simulink model "v2015a_Sensores"  (R2015a)
settings: Solver=ode45  SolverMode=SingleTasking  StartTime=0.0  StopTime=10.0  RelTol=1e-3
undefined symbols (not defined in the file): bias_mag, bias_sun, Eclipse, heading_mag, Mag_I, Pos_Sun_I, tilt_mag, v_I_S
libraries: simulink_extras x4, aerolibconvert2 x3, aerolibutil x2, aerolibtransform2 x2
settings Model: CovMetricSettings=dwe  CovHtmlReporting=off  covSaveCumulativeToWorkspaceVar=off  CovSaveSingleToWorkspaceVar=off  CovExternalEMLEnable=on  Creator=kakat  LastModifiedBy=kakat
settings DataIOCC: LimitDataPoints=off  SaveFormat=Dataset  ReturnWorkspaceOutputs=on
settings DebuggingCC: SFUnexpectedBacktrackingDiag=error  SFNoUnconditionalDefaultTransitionDiag=error
settings HardwareCC: ProdBitPerPointer=64  ProdLargestAtomicFloat=Float  ProdIntDivRoundTo=Zero  ProdEndianess=LittleEndian  ProdHWDeviceType=Specified
settings ModelReferenceCC: PropagateSignalLabelsOutOfModel=on
settings SFSimCC: SimUseLocalCustomCode=on
settings RTWCC: RTWUseLocalCustomCode=on
settings GRTTargetCC: TargetLangStandard=C99 (ISO)

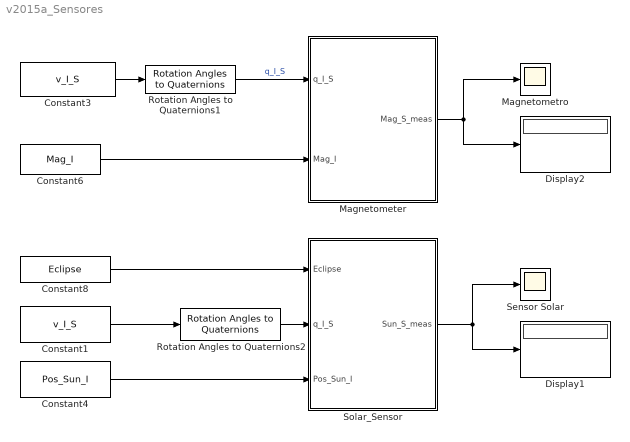
== system v2015a_Sensores ==
  Constant1 : Constant  Value=v_I_S
  Constant3 : Constant  Value=v_I_S
  Constant4 : Constant  Value=Pos_Sun_I
  Constant6 : Constant  Value=Mag_I
  Constant8 : Constant  Value=Eclipse
  Display1 : Display
  Display2 : Display
  Magnetometer : Subsystem
  Magnetometro : Scope
      settings: TimeRange=auto  MaxDataPoints=5000  SaveToWorkspace=off  YMin=-0.000045  YMax=0.000045  SampleTime=-1
  Rotation Angles to Quaternions1 : aerolibtransform2/Rotation Angles to Quaternions  rotationOrder=ZYX
  Rotation Angles to Quaternions2 : aerolibtransform2/Rotation Angles to Quaternions  rotationOrder=ZYX
  Sensor Solar : Scope
      settings: TimeRange=auto  MaxDataPoints=5000  SaveToWorkspace=off  SaveName=ScopeData  YMin=-182918141.73544  YMax=171344381.20005  SampleTime=-1
  Solar_Sensor : Subsystem
  wires:
  Constant3/1 -> Rotation Angles to Quaternions1/1
  Magnetometer/1(Mag_S_meas) -> Display2/1, Magnetometro/1
  Constant6/1 -> Magnetometer/2(Mag_I)
  Constant1/1 -> Rotation Angles to Quaternions2/1
  Rotation Angles to Quaternions2/1 -> Solar_Sensor/2(q_I_S)
  Solar_Sensor/1(Sun_S_meas) -> Display1/1, Sensor Solar/1
  Constant8/1 -> Solar_Sensor/1(Eclipse)
  Constant4/1 -> Solar_Sensor/3(Pos_Sun_I)
  Rotation Angles to Quaternions1/1 -> Magnetometer/1(q_I_S)  "q_I_S"

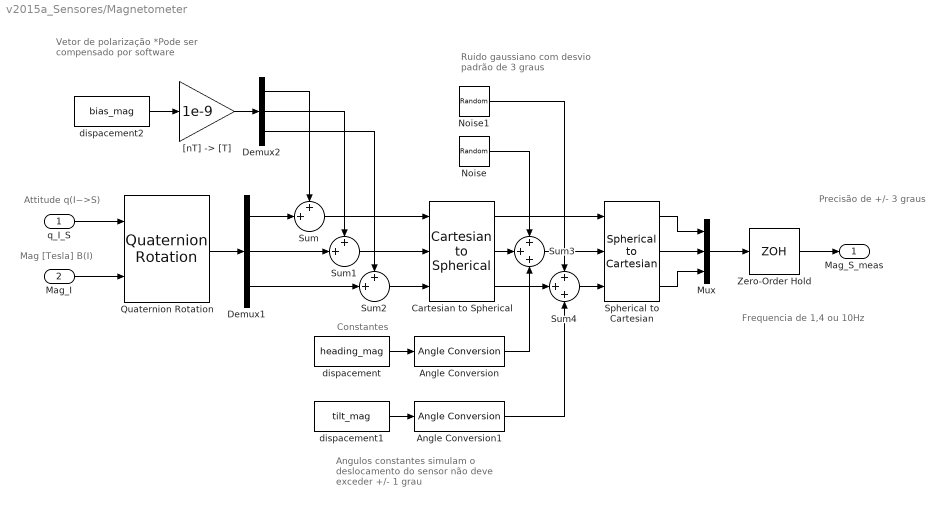
== system v2015a_Sensores/Magnetometer ==
  note: Attitude q(I−>S)
  note: Angulos constantes
      | simulam o deslocamento do sensor
      | não deve exceder +/- 1 grau
  note: Precisão de
      | +/- 3 graus
  note: Vetor de polarização
      | *Pode ser compensado
      | por software
  note: Frequencia de
      | 1,4 ou 10Hz
  note: Ruido gaussiano com
      | desvio padrão de 3 graus
  note: Constantes
  note: Mag [Tesla] B(I)
  q_I_S : Inport
  Mag_I : Inport  Port=2
  Angle Conversion : aerolibconvert2/Angle Conversion  IU=deg  OU=rad
  Angle Conversion1 : aerolibconvert2/Angle Conversion  IU=deg  OU=rad
  Cartesian to Spherical : simulink_extras/Transformations/Cartesian to Spherical
  Demux1 : Demux  Outputs=3
  Demux2 : Demux  Outputs=3
  Mux : Mux  Inputs=3
  Noise : RandomNumber  Variance=3  SampleTime=0.1
  Noise1 : RandomNumber  Variance=3  SampleTime=0.1
  Quaternion Rotation : aerolibutil/Quaternion Rotation
  Spherical to Cartesian : simulink_extras/Transformations/Spherical to Cartesian
  Sum : Sum  Inputs=++|
  Sum1 : Sum  Inputs=++|
  Sum2 : Sum  Inputs=++|
  Sum3 : Sum  Inputs=+++
  Sum4 : Sum  Inputs=+++
  Zero-Order Hold : ZeroOrderHold  SampleTime=.1
  "[nT] -> [T]" : Gain  Gain=1e-9
  dispacement : Constant  Value=heading_mag
  dispacement1 : Constant  Value=tilt_mag
  dispacement2 : Constant  Value=bias_mag
  Mag_S_meas : Outport
  wires:
  Quaternion Rotation/1 -> Demux1/1
  Mag_I/1 -> Quaternion Rotation/2
  Zero-Order Hold/1 -> Mag_S_meas/1
  Spherical to Cartesian/1 -> Mux/1
  Spherical to Cartesian/2 -> Mux/2
  dispacement1/1 -> Angle Conversion1/1
  Spherical to Cartesian/3 -> Mux/3
  Noise/1 -> Sum3/1
  Mux/1 -> Zero-Order Hold/1
  dispacement2/1 -> "[nT] -> [T]"/1
  dispacement/1 -> Angle Conversion/1
  Angle Conversion/1 -> Sum3/3
  Noise1/1 -> Sum4/1
  Demux1/1 -> Sum/2
  Angle Conversion1/1 -> Sum4/3
  q_I_S/1 -> Quaternion Rotation/1
  Cartesian to Spherical/2 -> Sum3/2
  Cartesian to Spherical/1 -> Spherical to Cartesian/1
  Sum3/1 -> Spherical to Cartesian/2
  Demux2/3 -> Sum2/1
  Sum4/1 -> Spherical to Cartesian/3
  Demux2/1 -> Sum/1
  Cartesian to Spherical/3 -> Sum4/2
  Demux1/3 -> Sum2/2
  Sum2/1 -> Cartesian to Spherical/3
  Sum/1 -> Cartesian to Spherical/1
  Demux1/2 -> Sum1/2
  Sum1/1 -> Cartesian to Spherical/2
  Demux2/2 -> Sum1/1
  "[nT] -> [T]"/1 -> Demux2/1

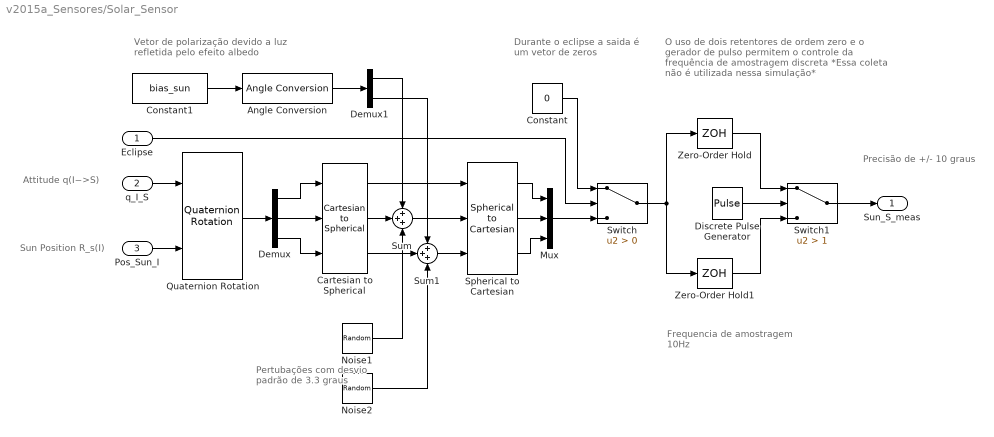
== system v2015a_Sensores/Solar_Sensor ==
  note: Sun Position R_s(I)
  note: O uso de dois retentores de ordem zero e o gerador de pulso permitem o controle da frequência de amostragem discreta
      |
      | *Essa coleta não é utilizada nessa simulação*
  note: Pertubações com desvio padrão de 3.3 graus
  note: Precisão de +/- 10 graus
  note: Vetor de polarização devido a luz refletida pelo efeito albedo
  note: Durante o eclipse a saida é um vetor de zeros
  note: Frequencia de amostragem 10Hz
  note: Attitude q(I−>S)
  Eclipse : Inport
  q_I_S : Inport  Port=2
  Pos_Sun_I : Inport  Port=3
  Angle Conversion : aerolibconvert2/Angle Conversion  IU=deg  OU=rad
  Cartesian to Spherical : simulink_extras/Transformations/Cartesian to Spherical
  Constant : Constant  Value=0
  Constant1 : Constant  Value=bias_sun
  Demux : Demux  Outputs=3
  Demux1 : Demux  Outputs=2
  Discrete Pulse Generator : DiscretePulseGenerator  Period=10  PulseWidth=5
  Mux : Mux  Inputs=3
  Noise1 : RandomNumber  SampleTime=0.1
  Noise2 : RandomNumber  SampleTime=0.1
  Quaternion Rotation : aerolibutil/Quaternion Rotation
  Spherical to Cartesian : simulink_extras/Transformations/Spherical to Cartesian
  Sum : Sum  Inputs=+++
  Sum1 : Sum  Inputs=+++
  Switch : Switch  Criteria=u2 > Threshold
      settings: LockScale=on
  Switch1 : Switch  Criteria=u2 > Threshold  Threshold=1
  Zero-Order Hold : ZeroOrderHold  SampleTime=0.1
  Zero-Order Hold1 : ZeroOrderHold  SampleTime=0.1
  Sun_S_meas : Outport
  wires:
  Angle Conversion/1 -> Demux1/1
  Constant1/1 -> Angle Conversion/1
  Sum1/1 -> Spherical to Cartesian/3
  Spherical to Cartesian/1 -> Mux/1
  Sum/1 -> Spherical to Cartesian/2
  Cartesian to Spherical/2 -> Sum/2
  Demux/3 -> Cartesian to Spherical/3
  Spherical to Cartesian/2 -> Mux/2
  Cartesian to Spherical/1 -> Spherical to Cartesian/1
  Quaternion Rotation/1 -> Demux/1
  Spherical to Cartesian/3 -> Mux/3
  Zero-Order Hold/1 -> Switch1/1
  Demux1/2 -> Sum1/1
  Noise1/1 -> Sum/3
  Switch1/1 -> Sun_S_meas/1
  Noise2/1 -> Sum1/3
  Switch/1 -> Zero-Order Hold1/1, Zero-Order Hold/1
  Eclipse/1 -> Switch/2
  Demux/2 -> Cartesian to Spherical/2
  Mux/1 -> Switch/3
  Demux/1 -> Cartesian to Spherical/1
  Demux1/1 -> Sum/1
  Zero-Order Hold1/1 -> Switch1/3
  Constant/1 -> Switch/1
  Discrete Pulse Generator/1 -> Switch1/2
  Cartesian to Spherical/3 -> Sum1/2
  Pos_Sun_I/1 -> Quaternion Rotation/2
  q_I_S/1 -> Quaternion Rotation/1
